simulink model "rt_ueb_s50"  (R2013a)
settings: Solver=ode45  StartTime=0.0  StopTime=100e-3  RelTol=1e-3
undefined symbols (not defined in the file or in its folder): a, KD, KI, Kp
settings Model: Creator=mainster  LastModifiedBy=mainster

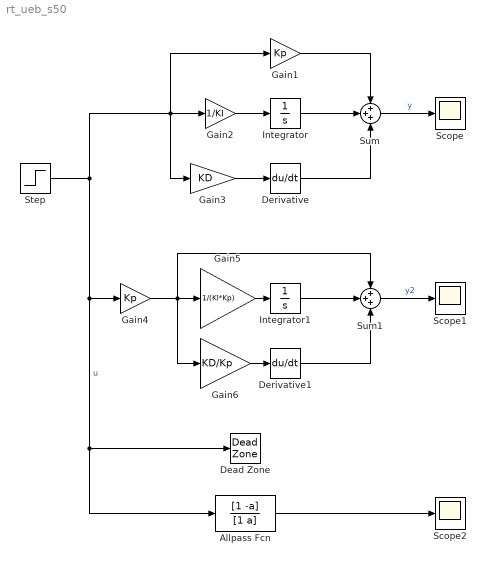
== system rt_ueb_s50 ==
  Allpass Fcn : TransferFcn  Numerator=[1 -a]  Denominator=[1 a]
  Dead Zone : DeadZone  SaturateOnIntegerOverflow=on
  Derivative : Derivative
  Derivative1 : Derivative
  Gain1 : Gain  Gain=Kp
  Gain2 : Gain  Gain=1/KI
  Gain3 : Gain  Gain=KD
  Gain4 : Gain  Gain=Kp
  Gain5 : Gain  Gain=1/(KI*Kp)
  Gain6 : Gain  Gain=KD/Kp
  Integrator : Integrator
  Integrator1 : Integrator
  Scope : Scope
  Scope1 : Scope
  Scope2 : Scope
      settings: SaveName=ScopeData2
  Step : Step  Time=10e-3  SampleTime=0
  Sum : Sum  Inputs=+++
  Sum1 : Sum  Inputs=+++
  wires:
  Step/1 -> Allpass Fcn/1, Dead Zone/1, Gain4/1, Gain1/1, Gain3/1, Gain2/1  "u"
  Gain1/1 -> Sum/1
  Integrator/1 -> Sum/2
  Gain3/1 -> Derivative/1
  Derivative/1 -> Sum/3
  Gain2/1 -> Integrator/1
  Gain4/1 -> Gain6/1, Gain5/1, Sum1/1
  Integrator1/1 -> Sum1/2
  Gain6/1 -> Derivative1/1
  Derivative1/1 -> Sum1/3
  Gain5/1 -> Integrator1/1
  Allpass Fcn/1 -> Scope2/1
  Sum1/1 -> Scope1/1  "y2"
  Sum/1 -> Scope/1  "y"
